simulink model "MATLAB_Exercise_5a"  (R2017b)
settings: Solver=FixedStepAuto  StartTime=0.0  StopTime=5.8  FixedStep=0.1  RelTol=1e-3
settings Model: Creator=chenjiasheng  LastModifiedBy=chenjiasheng

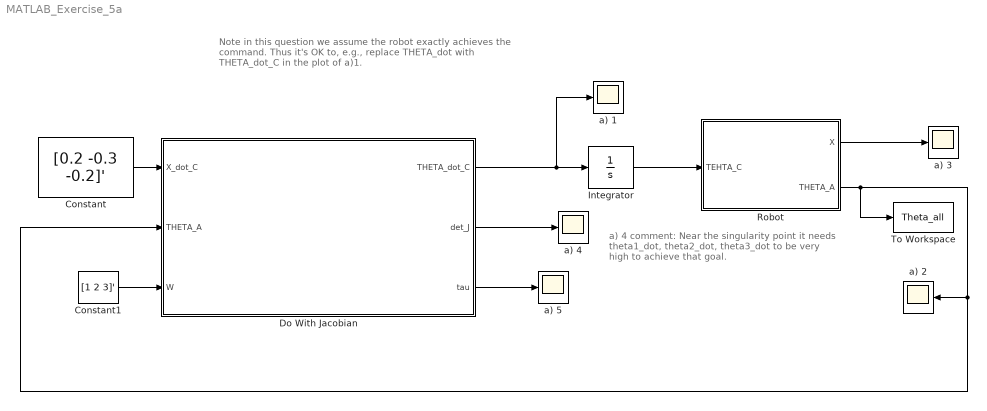
== system MATLAB_Exercise_5a ==
  note: Note in this question we assume the robot exactly achieves the command. Thus it's OK to, e.g., replace THETA_dot with THETA_dot_C in the plot of a)1.
  note: a) 4 comment: Near the singularity point it needs theta1_dot, theta2_dot, theta3_dot to be very high to achieve that goal.
  Constant : Constant  Value=[0.2 -0.3 -0.2]'
  Constant1 : Constant  Value=[1 2 3]'
  Do With Jacobian : MATLAB Function  TreatAsAtomicUnit=on
  Integrator : Integrator  InitialCondition=[pi/18 pi/9 pi/6]'
  Robot : MATLAB Function  TreatAsAtomicUnit=on
  To Workspace : ToWorkspace  VariableName=Theta_all  SampleTime=0.1
  a) {1..5} (5 alike) : Scope
  wires:
  Constant/1 -> Do With Jacobian/1(X_dot_C)
  Do With Jacobian/1(THETA_dot_C) -> a) 1/1, Integrator/1
  Integrator/1 -> Robot/1(TEHTA_C)
  Robot/2(THETA_A) -> To Workspace/1, a) 2/1, Do With Jacobian/2(THETA_A)
  Robot/1(X) -> a) 3/1
  Do With Jacobian/2(det_J) -> a) 4/1
  Constant1/1 -> Do With Jacobian/3(W)
  Do With Jacobian/3(tau) -> a) 5/1

== matlab function MATLAB_Exercise_5a/Robot ==
  data: X output; TEHTA_C input; THETA_A output
function [X,THETA_A] = Robot(TEHTA_C)
L1=4;
L2=3;
L3=2;
THETA_A = TEHTA_C;
theta1=THETA_A(1);
theta2=THETA_A(2);
theta3=THETA_A(3);
x=L1*cos(theta1)+L2*cos(theta1+theta2)+L3*cos(theta1+theta2+theta3)
y=L1*sin(theta1)+L2*sin(theta1+theta2)+L3*sin(theta1+theta2+theta3)
phi=theta1+theta2+theta3;
X=[x y phi]'
end

== matlab function MATLAB_Exercise_5a/Do With Jacobian ==
  data: X_dot_C input; THETA_dot_C output; THETA_A input; det_J output; W input; tau output
function [THETA_dot_C,det_J,tau]= fcn(X_dot_C,THETA_A,W)
L1=4
L2=3
L3=2
theta1=THETA_A(1)
theta2=THETA_A(2)
theta3=THETA_A(3)
J=[-L1*sin(theta1)-L2*sin(theta1+theta2)-L3*sin(theta1+theta2+theta3) -L2*sin(theta1+theta2)-L3*sin(theta1+theta2+theta3) -L3*sin(theta1+theta2+theta3);
    L1*cos(theta1)+L2*cos(theta1+theta2)+L3*cos(theta1+theta2+theta3)  L2*cos(theta1+theta2)+L3*cos(theta1+theta2+theta3)  L3*cos(theta1+theta2+theta3);
    1                                                                  1                                                   1];
THETA_dot_C=inv(J)*X_dot_C
det_J=det(J)
tau=J'*W
end
